simulink model "MPPTModel"  (R2022a)
settings: Solver=VariableStepAuto  StartTime=0.0  StopTime=10  RelTol=1e-3
model workspace (MAT data in the model file):
  Volts = Simulink.Signal
  Volts.DataType = 'double'
  Volts.Dimensions = -1
  Volts.DimensionsMode = 'auto'
  Volts.Complexity = 'auto'
  Volts.SampleTime = -1
  Volts.SamplingMode = 'auto'
libraries: spsSeriesRLCBranchLib x5, dsparch4 x4, spsVoltageMeasurementLib x3, spsCurrentMeasurementLib x2, spsPVArrayLib x2, spsDiodeLib x1, spsMosfetLib x1, simulink x1, spspowerguiLib x1
settings Model: Creator=burmesdani  LastModifiedBy=ian
settings SolverCC: AlgebraicLoopSolver=TrustRegion
settings DebuggingCC: UnconnectedInputMsg=warning  UnconnectedOutputMsg=warning  UnconnectedLineMsg=warning  SFMachineParentedDataDiag=warning
settings RTWCC: DLArmComputeVersion=19.05

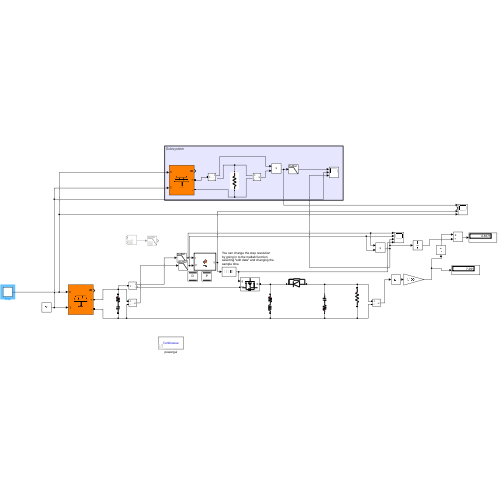
[thumbnail: Simulink's stored preview of the top-level diagram]
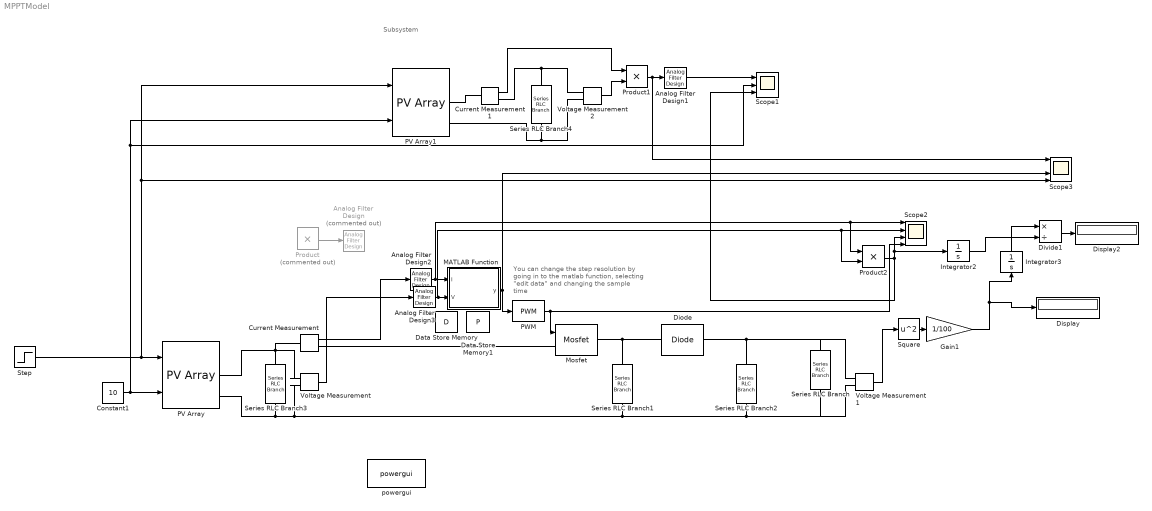
== system MPPTModel ==
  note: Subsystem
  note: You can change the step resolution by going in to the matlab function, selecting "edit data" and changing the sample time
  Analog Filter Design : dsparch4/Analog Filter Design  Commented=on  method=Butterworth  filttype=Lowpass  N=4  Wlo=30  Whi=80  Rp=2  Rs=40
  Analog Filter Design1 : dsparch4/Analog Filter Design  method=Butterworth  filttype=Lowpass  N=4  Wlo=30  Whi=80  Rp=2  Rs=40
  Analog Filter Design2 : dsparch4/Analog Filter Design  method=Butterworth  filttype=Lowpass  N=4  Wlo=30  Whi=80  Rp=2  Rs=40
  Analog Filter Design3 : dsparch4/Analog Filter Design  method=Butterworth  filttype=Lowpass  N=4  Wlo=30  Whi=80  Rp=2  Rs=40
  Constant1 : Constant  Value=10
  Current Measurement : spsCurrentMeasurementLib/Current Measurement  PhasorSimulation=off  OutputType=Complex  PSBequivalent=0
  Current Measurement1 : spsCurrentMeasurementLib/Current Measurement  PhasorSimulation=off  OutputType=Complex  PSBequivalent=0
  Data Store Memory : DataStoreMemory  DataStoreName=D  ReadBeforeWriteMsg=warning  WriteAfterWriteMsg=warning  WriteAfterReadMsg=warning  ShowAdditionalParam=off  OutDataTypeStr=double
  Data Store Memory1 : DataStoreMemory  DataStoreName=P  ReadBeforeWriteMsg=warning  WriteAfterWriteMsg=warning  WriteAfterReadMsg=warning  ShowAdditionalParam=off  OutDataTypeStr=double
  Diode : spsDiodeLib/Diode  Ron=0.001  Lon=0  Vf=0.8  IC=0  UseSnubber=0  Rs=500  Cs=250e-9  Measurements=off
  Display : Display
  Display2 : Display
  Divide1 : Product  Inputs=*/
  Gain1 : Gain  Gain=1/100
  Integrator2 : Integrator
  Integrator3 : Integrator
  MATLAB Function : MATLAB Function  TreatAsAtomicUnit=on
  Mosfet : spsMosfetLib/Mosfet  Ron=0.1  Lon=0  Rd=0.001  Vfd=0  IC=0  Rs=1e5  Cs=inf  Measurements=off
  PV Array : spsPVArrayLib/PV Array  Npar=2  Nser=1  PlotType=array @ 1000 W/m2 & specified temperatures  S_vec="[ 1000  500  100 ]"  Temp_C_vec="[ 45 25  ]"  ModuleName=User-defined  PlotWhenSelected=off  Pm=9.918  Ncell=36  Voc=21.8  Isc=0.61  Vm=17.4  Im=0.57  beta_Voc_pc=-0.36099  alpha_Isc_pc=0.102  beta_Voc=-0.078696  alpha_Isc=0.0006222  IL=0.61135  I0=2.2733e-11  nI=0.98214  Rsh=2141.245  Rs=3.0779  RobustModel=off  RobustCellTemperature=313.3991  BAL=on  Tc=1e-6  Tfilter=5e-5
  PV Array1 : spsPVArrayLib/PV Array  Npar=1  Nser=2  PlotType=array @ 1000 W/m2 & specified temperatures  S_vec="[ 1000  500  100 ]"  Temp_C_vec="[ 45 25  ]"  ModuleName=User-defined  PlotWhenSelected=off  Pm=9.918  Ncell=36  Voc=21.8  Isc=0.61  Vm=17.4  Im=0.57  beta_Voc_pc=-0.36099  alpha_Isc_pc=0.102  beta_Voc=-0.078696  alpha_Isc=0.0006222  IL=0.61135  I0=2.2733e-11  nI=0.98214  Rsh=2141.245  Rs=3.0779  RobustModel=off  RobustCellTemperature=313.3991  BAL=on  Tc=1e-6  Tfilter=5e-5
  PWM : simulink/Discontinuities/PWM  DisableCoverage=on  Period=1/30000  DisallowZeroDutyCycle=off  RunAtFixedTimeIntervals=off  SampleTime=0.1
  Product : Product  Commented=on
  Product1 : Product
  Product2 : Product
  Scope1 : Scope  NumInputPorts=3
  Scope2 : Scope  NumInputPorts=4
  Scope3 : Scope  NumInputPorts=4
  Series RLC Branch : spsSeriesRLCBranchLib/Series RLC Branch  LConnTagsString=__new0  RConnTagsString=__new0  BranchType=R  Resistance=100  Inductance=1e-3  SetiL0=off  InitialCurrent=0  Capacitance=1e-6  Setx0=off  InitialVoltage=0  Measurements=None
  Series RLC Branch1 : spsSeriesRLCBranchLib/Series RLC Branch  LConnTagsString=__new0  RConnTagsString=__new0  BranchType=RL  Resistance=0.00002  Inductance=0.0015  SetiL0=off  InitialCurrent=0  Capacitance=1e-6  Setx0=off  InitialVoltage=0  Measurements=None
  Series RLC Branch2 : spsSeriesRLCBranchLib/Series RLC Branch  LConnTagsString=__new0  RConnTagsString=__new0  BranchType=RC  Resistance=0.00002  Inductance=1e-3  SetiL0=off  InitialCurrent=0  Capacitance=4.8e-6  Setx0=off  InitialVoltage=0  Measurements=None
  Series RLC Branch3 : spsSeriesRLCBranchLib/Series RLC Branch  LConnTagsString=__new0  RConnTagsString=__new0  BranchType=RC  Resistance=0.00002  Inductance=1e-3  SetiL0=off  InitialCurrent=0  Capacitance=100e-6  Setx0=off  InitialVoltage=0  Measurements=None
  Series RLC Branch4 : spsSeriesRLCBranchLib/Series RLC Branch  LConnTagsString=__new0  RConnTagsString=__new0  BranchType=R  Resistance=100  Inductance=1e-3  SetiL0=off  InitialCurrent=0  Capacitance=1e-6  Setx0=off  InitialVoltage=0  Measurements=None
  Square : Math  Operator=square
  Step : Step  Time=0.5  After=400  SampleTime=0
  Voltage Measurement : spsVoltageMeasurementLib/Voltage Measurement  PhasorSimulation=off  OutputType=Complex  PSBequivalent=0
  Voltage Measurement1 : spsVoltageMeasurementLib/Voltage Measurement  PhasorSimulation=off  OutputType=Complex  PSBequivalent=0
  Voltage Measurement2 : spsVoltageMeasurementLib/Voltage Measurement  PhasorSimulation=off  OutputType=Complex  PSBequivalent=0
  powergui : spspowerguiLib/powergui  Priority=1  SimulationMode=Continuous  SampleTime=50e-6  frequency=60  Iterations=50  frequencyindice=0  Pbase=100e6  ErrMax=1e-4  UnitsV=kV  UnitsW=MW  buscounter=0  FunctionMessages=off  echomessages=off  EnableUseOfTLC=off  CurrentSourceSwitches=off  DisableSnubberDevices=off  DisableRonSwitches=off  DisableVfSwitches=off  DisplayEquations=off  AutomaticDiscreteSolvers=off  SolverType=Tustin/Backward Euler (TBE)  Interpol=off  ExternalGateDelay=off  methode=off  Ts=100  x0status=blocks  SPID=on  SwTol=0  HookPort=off  NonlinearTolerance=1e-4  nMaxIteration=100  ContinueOnMaxIteration=off  RestoreLinks=warning  ResistiveCurrentMeasurement=off  Frange=[0:2:500]  Ylog=off  Xlog=on  ShowGrid=off  save=off  variable=ZData  structure=0  ZoomFFT=off  StartTime=0.0  cycles=1  DisplayStyle=1  fundamental=60  FreqAxis=off  MaxFrequency=1000  frequencyindicesteady=1  RmsSteady=1  display=off
  wires:
  PWM/1 -> Mosfet/1, Scope2/4
  MATLAB Function/1(y) -> Scope3/3, PWM/1
  Voltage Measurement1/1 -> Square/1
  Square/1 -> Gain1/1
  Voltage Measurement/1 -> Analog Filter Design3/1
  Constant1/1 -> PV Array/2, Scope1/2, PV Array1/2
  Current Measurement1/1 -> Product1/1
  Voltage Measurement2/1 -> Product1/2
  Step/1 -> Scope3/4, PV Array1/1, PV Array/1
  Product1/1 -> Scope3/1, Analog Filter Design1/1
  Analog Filter Design1/1 -> Scope1/1
  Gain1/1 -> Display/1, Integrator3/1
  Product/1 -> Analog Filter Design/1
  Current Measurement/1 -> Analog Filter Design2/1
  Product2/1 -> Scope2/3, Integrator2/1, Scope1/3
  Divide1/1 -> Display2/1
  Integrator3/1 -> Divide1/1
  Integrator2/1 -> Divide1/2
  Analog Filter Design2/1 -> Product2/1, Scope2/1, MATLAB Function/1(I)
  Analog Filter Design3/1 -> Product2/2, Scope2/2, MATLAB Function/2(V)
  connections:
  PV Array/RConn2 -- Series RLC Branch3/RConn1 -- Series RLC Branch/RConn1 -- Voltage Measurement1/LConn2 -- Series RLC Branch2/LConn1 -- Series RLC Branch1/RConn1 -- Voltage Measurement/LConn2
  PV Array/RConn1 -- Series RLC Branch3/LConn1 -- Voltage Measurement/LConn1 -- Current Measurement/LConn1
  Series RLC Branch1/LConn1 -- Diode/RConn1 -- Mosfet/RConn1
  Series RLC Branch2/RConn1 -- Voltage Measurement1/LConn1 -- Series RLC Branch/LConn1 -- Diode/LConn1
  Current Measurement/RConn1 -- Mosfet/LConn1
  Series RLC Branch4/RConn1 -- Voltage Measurement2/LConn2 -- PV Array1/RConn2
  Current Measurement1/LConn1 -- PV Array1/RConn1
  Current Measurement1/RConn1 -- Voltage Measurement2/LConn1 -- Series RLC Branch4/LConn1

== matlab function MPPTModel/MATLAB Function ==
  settings: updateMethod=DISCRETE  sampleTime=0.1
  data: y output; D data_store_memory; P data_store_memory; I input; V input
function y  = fcn(I, V)

%declare global variables (presistent) and assign values
persistent Dprev Vprev Iprev;
if isempty(Dprev)
    %duty cycle value calculated in section 3.1.1.2
    Dinit = 0.7259;
    Vprev = 0;
    Iprev = 0;
    Dprev = Dinit; 
end
%small change duty cycle 
%observe the sensor values
inc = 0.0025;
dV = V - Vprev;
dI = I - Iprev;
if dV == 0
    if dI == 0
        D = Dprev;
    else
        if dI > 0
            D = Dprev - (inc); %parameter met for decreasing duty cycle
        else
            D = Dprev + (inc); %parameter met for increasing duty cycle 
        end
    end
else
    if dI/dV == -I/V
        D = Dprev;
    else
        if dI/dV > -I/V
            D = Dprev - (inc); %parameter met for decreasing duty cycle
        else
            D = Dprev + (inc); %parameter met for increasing duty cycle
        end
    end
end
%reassign previous values to current values
Dprev = D;
Vprev = V;
Iprev = I;
%output to the simulated gate drive
y = D;
